simulink model "sampleModel170"  (R2021b)
settings: Solver=VariableStepAuto  StartTime=0.0  StopTime=10.0  RelTol=1e-3
libraries: simulink x5, slpidlib x1
settings Model: Creator=user  LastModifiedBy=user

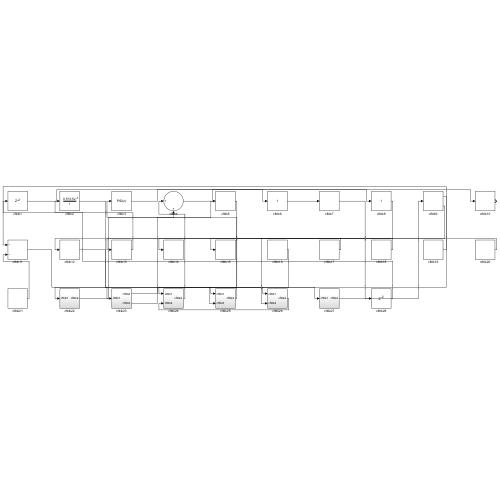
[thumbnail: Simulink's stored preview of the top-level diagram]
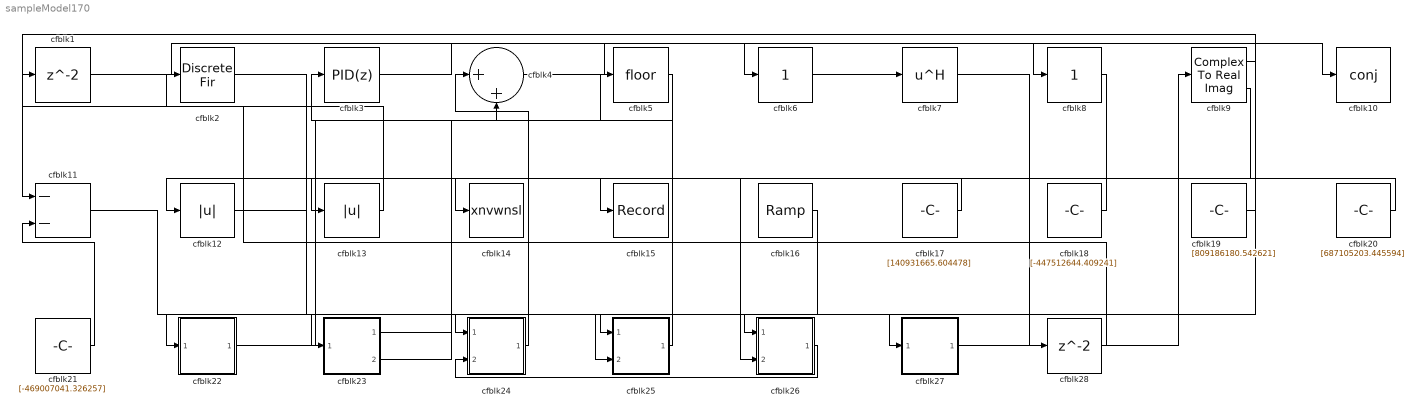
== system sampleModel170 ==
  cfblk1 : Delay  SampleTime=1
  cfblk10 : Math  Operator=conj  SaturateOnIntegerOverflow=on
  cfblk11 : Sum  Inputs=--
  cfblk12 : Abs
  cfblk13 : Abs
  cfblk14 : ToWorkspace  VariableName=xnvwnsl  SaveFormat=Timeseries  SampleTime=-1
  cfblk15 : Record  FileSettingsInternal="{\"entries\":[{\"content\":{\"excelSettings\":{\"content\":{},\"type\":\"Streamout.ExcelSettings\"}},\"type\":\"Streamout.FileSettingStorage\",\"uuid\":\"54ea01bb-11ee-411b-9db7-375307b2bc9b\"}],\"packageUris\":[\"http://schema.mathworks.com/mf0/streamout_blocks/R2020a\"],\"version\":\"1.0\"}"  SignalsInternal="{\"entries\":[{\"content\":{\"signals\":[{\"content\":{\"blockPath\":[\"sampleModel170/cfblk15\"],\"channel\":[],\"dimensions\":[1],\"domain\":\"sampleModel170/cfblk15\",\"lineColor\":\"#22b573\",\"plots\":[1],\"port\":1,\"sid\":[\"\"],\"signalID\":6353,\"signalName\":\"cfblk8\"},\"type\":\"RecordBlkView.Signal\",\"uuid\":\"c27c39d6-17b0-4d17-8c05-65d208e17416\"}]},\"type\":\"RecordBlkView.InputSignals\",\"uuid\":\"905179ff-a989-4d47-ae26-5f4de0177f01\"}],\"packageUris\":[\"http://schema.mathworks.com/mf0/streamout_blocks/R2020a\"],\"version\":\"1.0\"}"  VisualizationBindings="{\"sparklinesplugin\":{\"info\":[{\"bindingParametersList\":[],\"subplotID\":1}]}}"
  cfblk16 : simulink/Sources/Ramp  slope=[9008.312109]  start=[18.162069]  InitialOutput=[966180.336838]
  cfblk17 : Constant  Value=[140931665.604478]  SampleTime=1
  cfblk18 : Constant  Value=[-447512644.409241]  SampleTime=1
  cfblk19 : Constant  Value=[809186180.542621]  SampleTime=1
  cfblk2 : DiscreteFir  SampleTime=1
  cfblk20 : Constant  Value=[687105203.445594]  SampleTime=1
  cfblk21 : Constant  Value=[-469007041.326257]  SampleTime=1
  cfblk22 : Subsystem
  cfblk23 : Subsystem
  cfblk24 : Subsystem
  cfblk25 : Subsystem
  cfblk26 : Subsystem
  cfblk27 : Subsystem
  cfblk28 : Delay  SampleTime=1
  cfblk3 : slpidlib/PID Controller  Controller=PID  Form=Parallel  TimeDomain=Discrete-time  UseExternalTs=off  SampleTime=1  IntegratorMethod=Forward Euler  FilterMethod=Forward Euler  ControllerParametersSource=internal  P=1  I=1  D=0  UseFilter=on  N=100  TunerSelectOption=Transfer Function Based (PID Tuner App)  InitialConditionSource=internal  InitialConditionForIntegrator=0  InitialConditionForFilter=0  DifferentiatorICPrevScaledInput=0  ExternalReset=none  TrackingMode=off  Kt=1  LimitOutput=off  SatLimitsSource=internal  UpperSaturationLimit=inf  LowerSaturationLimit=-inf  LinearizeAsGain=off  AntiWindupMode=none  Kb=1  POutMin=[]  POutMax=[]  IOutMin=[]  IOutMax=[]  DOutMin=[]  DOutMax=[]  NOutMin=[]  NOutMax=[]  SumOutMin=[]  SumOutMax=[]  SaturationOutMin=[]  SaturationOutMax=[]  PParamMin=[]  PParamMax=[]  IParamMin=[]  IParamMax=[]  DParamMin=[]  DParamMax=[]  NParamMin=[]  NParamMax=[]  KbParamMin=[]  KbParamMax=[]  KtParamMin=[]  KtParamMax=[]  KbOutMin=[]  KbOutMax=[]  KtOutMin=[]  KtOutMax=[]  IntegratorOutMin=[]  IntegratorOutMax=[]  FilterOutMin=[]  FilterOutMax=[]  SumI1OutMin=[]  SumI1OutMax=[]  SumI2OutMin=[]  SumI2OutMax=[]  SumI3OutMin=[]  SumI3OutMax=[]  SumI4OutMin=[]  SumI4OutMax=[]  SumDOutMin=[]  SumDOutMax=[]  DifferentiatorOutMin=[]  DifferentiatorOutMax=[]  FilterDiffOutCoefMin=[]  FilterDiffOutCoefMax=[]  ReciprocalOutMin=[]  ReciprocalOutMax=[]  SumDenOutMin=[]  SumDenOutMax=[]  SumNumOutMin=[]  SumNumOutMax=[]  DivideOutMin=[]  DivideOutMax=[]  UdiffTsProdOutMin=[]  UdiffTsProdOutMax=[]  NTsProdOutMin=[]  NTsProdOutMax=[]  UintegralTsProdOutMin=[]  UintegralTsProdOutMax=[]  UngainTsProdOutMin=[]  UngainTsProdOutMax=[]  IntegratorContinuousStateAttributes=''  IntegratorStateMustResolveToSignalObject=off  IntegratorRTWStateStorageClass=Auto  FilterContinuousStateAttributes=''  FilterStateMustResolveToSignalObject=off  FilterRTWStateStorageClass=Auto  ParallelPVariant=InternalParameters  IdealPVariant=Disabled  IVariant=InternalParameters  DVariant=InternalParameters  IntegratorVariant=Discrete  SatVariant=Disabled  AWVariant=Passthrough  PCopyVariant=Disabled  TRVariant=Disabled  FdbkBlocksVariant=Forward  IdealPFdbkVariant=Disabled  SatFdbkVariant=Disabled  DerivativeFilterVariant=ForwardEulerFilter  NVariant=InternalParameters  NCopyVariant=Disabled  FilterICVariant=InternalICsFilter  IntegratorICVariant=InternalICs  ExternalResetVariant=Disabled  TRSumVariant=Passthrough  SumFdbkVariant=Disabled  SumVariant=Sum_PID  TsampFilterVariant=InternalTs  TsampNgainVariant=Passthrough  TsampIntegralVariant=Passthrough  ExternalSaturationOutDataTypeStr=Inherit: Same as second input
  cfblk4 : Sum  Inputs=|++
  cfblk5 : Rounding
  cfblk6 : simulink/Math Operations/Slider Gain  gain=1  low=0  high=2
  cfblk7 : Math  Operator=hermitian  SaturateOnIntegerOverflow=on
  cfblk8 : simulink/Math Operations/Slider Gain  gain=1  low=0  high=2
  cfblk9 : ComplexToRealImag
  wires:
  cfblk24/1(cfblk2) -> cfblk4/1
  cfblk22/1(cfblk2) -> cfblk4/2
  cfblk18/1 -> cfblk14/1
  cfblk4/1 -> cfblk8/1
  cfblk27/1(cfblk2) -> cfblk9/1
  cfblk19/1 -> cfblk11/1
  cfblk5/1 -> cfblk24/1(cfblk1)
  cfblk1/1 -> cfblk10/1
  cfblk20/1 -> cfblk13/1
  cfblk17/1 -> cfblk12/1
  cfblk26/1(cfblk2) -> cfblk24/2(cfblk4)
  cfblk11/1 -> cfblk23/1(cfblk1)
  cfblk8/1 -> cfblk15/1
  cfblk6/1 -> cfblk7/1
  cfblk25/1(cfblk2) -> cfblk3/1
  cfblk2/1 -> cfblk27/1(cfblk1)
  cfblk13/1 -> cfblk1/1
  cfblk23/1(cfblk2) -> cfblk25/1(cfblk1)
  cfblk21/1 -> cfblk11/2
  cfblk16/1 -> cfblk22/1(cfblk1)
  cfblk23/2(cfblk3) -> cfblk5/1
  cfblk3/1 -> cfblk6/1
  cfblk12/1 -> cfblk26/1(cfblk1)
  cfblk9/1 -> cfblk25/2(cfblk3)
  cfblk9/2 -> cfblk26/2(cfblk4)
  cfblk7/1 -> cfblk28/1
  cfblk28/1 -> cfblk2/1

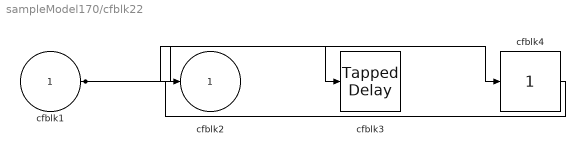
== system sampleModel170/cfblk22 ==
  cfblk1 : Inport
  cfblk3 : simulink/Discrete/Tapped Delay  vinit=0.0  samptime=-1  NumDelays=1  DelayOrder=Oldest  includeCurrent=off
  cfblk4 : simulink/Math Operations/Slider Gain  gain=1  low=0  high=2
  cfblk2 : Outport
  wires:
  cfblk1/1 -> cfblk4/1, cfblk3/1
  cfblk4/1 -> cfblk2/1

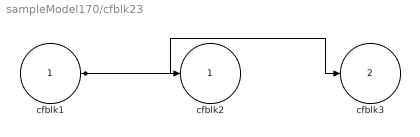
== system sampleModel170/cfblk23 ==
  cfblk1 : Inport
  cfblk2 : Outport
  cfblk3 : Outport  Port=2
  wires:
  cfblk1/1 -> cfblk3/1, cfblk2/1

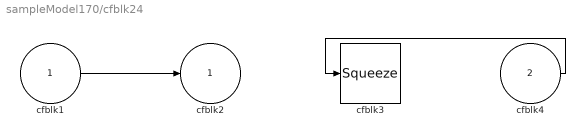
== system sampleModel170/cfblk24 ==
  cfblk1 : Inport
  cfblk4 : Inport  Port=2
  cfblk3 : Squeeze
  cfblk2 : Outport
  wires:
  cfblk1/1 -> cfblk2/1
  cfblk4/1 -> cfblk3/1

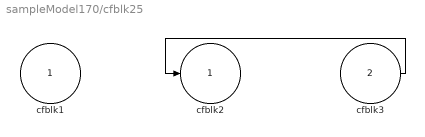
== system sampleModel170/cfblk25 ==
  cfblk1 : Inport
  cfblk3 : Inport  Port=2
  cfblk2 : Outport
  wires:
  cfblk3/1 -> cfblk2/1

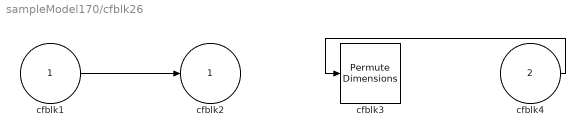
== system sampleModel170/cfblk26 ==
  cfblk1 : Inport
  cfblk4 : Inport  Port=2
  cfblk3 : PermuteDimensions
  cfblk2 : Outport
  wires:
  cfblk1/1 -> cfblk2/1
  cfblk4/1 -> cfblk3/1

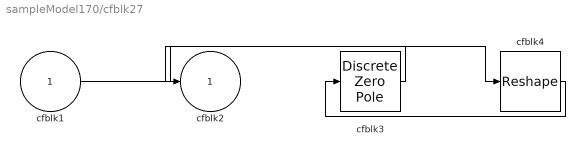
== system sampleModel170/cfblk27 ==
  cfblk1 : Inport
  cfblk3 : DiscreteZeroPole  Poles=[0 0.5]  Gain=1
  cfblk4 : Reshape
  cfblk2 : Outport
  wires:
  cfblk1/1 -> cfblk4/1
  cfblk4/1 -> cfblk3/1
  cfblk3/1 -> cfblk2/1
